simulink model "a7nl_sw_ged_ext_lsg"  (R2020b)
settings: Solver=ode45  StartTime=0.0  StopTime=40.0  MaxStep=0.01  RelTol=1e-3  EnableMultiTasking=on
model workspace (MAT data in the model file):
  A = 3
  c = 0.1
  delta = 0.1
  k = 1
  lambda = 0.2
  m = 2
  v0 = 0
  y0 = 2
settings Model: Creator=Reichl  LastModifiedBy=jakob
settings DataIOCC: LimitDataPoints=on  SaveFormat=Array  SignalLoggingSaveFormat=ModelDataLogs  ReturnWorkspaceOutputs=off
settings OptimizationCC: ExpressionDepthLimit=2147483647  LifeSpan=inf
settings DebuggingCC: UnderspecifiedInitializationDetection=Classic  MergeDetectMultiDrivingBlocksExec=none  SolverPrmCheckMsg=warning  FcnCallInpInsideContextMsg=warning  StateNameClashWarn=warning  SFUnexpectedBacktrackingDiag=warning  SFNoUnconditionalDefaultTransitionDiag=warning  SFExecutionAtInitializationDiag=none  ArithmeticOperatorsInVariantConditions=warning
settings HardwareCC: ProdBitPerPointer=32  ProdBitPerSizeT=32  ProdBitPerPtrDiffT=32  ProdLargestAtomicFloat=None  ProdIntDivRoundTo=Undefined  ProdEndianess=Unspecified  ProdWordSize=32  ProdHWDeviceType=32-bit Generic
settings ModelReferenceCC: PropagateSignalLabelsOutOfModel=off
settings SFSimCC: SimUseLocalCustomCode=off  CustomCodeUndefinedFunction=UseInterfaceOnly
settings RTWCC: RTWUseLocalCustomCode=off
settings CodeAppCC: StateflowObjectComments=on
settings GRTTargetCC: TargetLangStandard=C89/C90 (ANSI)  CombineOutputUpdateFcns=off  GRTInterface=on
settings ConfigComp: CovMetricSettings=dw  CovSaveCumulativeToWorkspaceVar=on  CovSaveSingleToWorkspaceVar=on  CovExternalEMLEnable=off  CovSFcnEnable=off

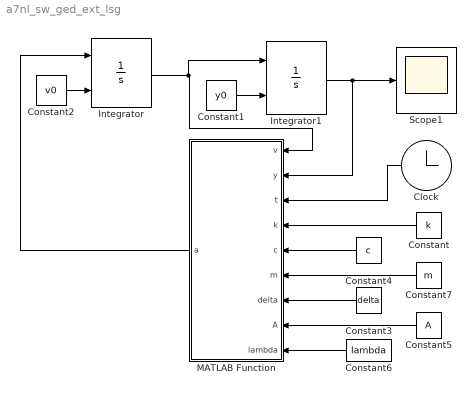
== system a7nl_sw_ged_ext_lsg ==
  Clock : Clock
  Constant : Constant  Value=k
  Constant1 : Constant  Value=y0
  Constant2 : Constant  Value=v0
  Constant3 : Constant  Value=delta
  Constant4 : Constant  Value=c
  Constant5 : Constant  Value=A
  Constant6 : Constant  Value=lambda
  Constant7 : Constant  Value=m
  Integrator : Integrator  InitialConditionSource=external
  Integrator1 : Integrator  InitialConditionSource=external  InitialCondition=3
  MATLAB Function : MATLAB Function  TreatAsAtomicUnit=on
  Scope1 : Scope
  wires:
  Integrator/1 -> Integrator1/1, MATLAB Function/1(v)
  Constant2/1 -> Integrator/2
  Constant1/1 -> Integrator1/2
  Integrator1/1 -> Scope1/1, MATLAB Function/2(y)
  MATLAB Function/1(a) -> Integrator/1
  Clock/1 -> MATLAB Function/3(t)
  Constant/1 -> MATLAB Function/4(k)
  Constant4/1 -> MATLAB Function/5(c)
  Constant3/1 -> MATLAB Function/7(delta)
  Constant5/1 -> MATLAB Function/8(A)
  Constant6/1 -> MATLAB Function/9(lambda)
  Constant7/1 -> MATLAB Function/6(m)

== matlab function a7nl_sw_ged_ext_lsg/MATLAB Function ==
  data: v input; a output; y input; t input; k input; c input; m input; delta input; A input; lambda input
function a = fcn(v,y,t,k,c,m,delta,A,lambda)

a = -2*delta*v - k/m*y - c/m*y^3 + ...
    A*exp(-lambda*t);
